simulink model "ideal_forward_converter"  (R2018a)
settings: Solver=FixedStepDiscrete  StartTime=0.0  StopTime=0.01  FixedStep=1e-08  RelTol=1e-3
libraries: powerlib x12, pePowerMeasurement x1
settings Model: Creator=gizemlikaradenizli61  LastModifiedBy=anılcanbudak
settings SolverCC: AlgebraicLoopSolver=LineSearch

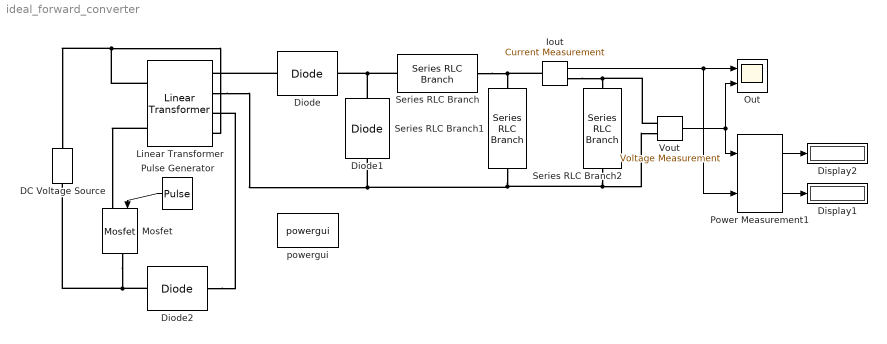
== system ideal_forward_converter ==
  DC Voltage Source : powerlib/Electrical Sources/DC Voltage Source  Amplitude=24  Measurements=None
  Diode : powerlib/Power Electronics/Diode  Ron=0.0001  Lon=0  Vf=0  IC=0  UseSnubber=0  Rs=500  Cs=250e-09  Measurements=off
  Diode1 : powerlib/Power Electronics/Diode  Ron=0.0001  Lon=0  Vf=0  IC=0  UseSnubber=0  Rs=500  Cs=250e-9  Measurements=off
  Diode2 : powerlib/Power Electronics/Diode  Ron=0.001  Lon=0  Vf=0  IC=0  UseSnubber=0  Rs=500  Cs=250e-9  Measurements=off
  Display1 : Display
  Display2 : Display
  Iout : powerlib/Measurements/Current Measurement  PhasorSimulation=off  OutputType=Complex  PSBequivalent=0
  Linear Transformer : powerlib/Elements/Linear Transformer  UNITS=SI  NominalPower=[ 40 30000]  winding1=[32 0.015 0]  winding2=[28.985 0.021 0]  ThreeWindings=on  winding3=[32 0.005 0]  RmLm=[500 0]  Measurements=None  DataType=on
  Mosfet : powerlib/Power Electronics/Mosfet  Ron=0.1  Lon=0  Rd=0.01  Vfd=0  IC=0  Rs=1e05  Cs=inf  Measurements=off
  Out : Scope  NumInputPorts=2
  Power Measurement1 : pePowerMeasurement/Power Measurement  OverrideUsingVariant=Discrete  F=30000  K=[0 1 2 3]  Ts=0.000001
  Pulse Generator : DiscretePulseGenerator  PulseType=Time based  Period=0.000033  PulseWidth=46
  Series RLC Branch : powerlib/Elements/Series RLC Branch  LConnTagsString=__new0  RConnTagsString=__new0  BranchType=L  Resistance=1  Inductance=5e-4  SetiL0=off  InitialCurrent=0  Capacitance=1e-6  Setx0=off  InitialVoltage=0  Measurements=None
  Series RLC Branch1 : powerlib/Elements/Series RLC Branch  LConnTagsString=__new0  RConnTagsString=__new0  BranchType=C  Resistance=1  Inductance=1e-3  SetiL0=off  InitialCurrent=0  Capacitance=10e-6  Setx0=off  InitialVoltage=0  Measurements=None
  Series RLC Branch2 : powerlib/Elements/Series RLC Branch  LConnTagsString=__new0  RConnTagsString=__new0  BranchType=R  Resistance=2.5  Inductance=1e-3  SetiL0=off  InitialCurrent=0  Capacitance=1e-6  Setx0=off  InitialVoltage=0  Measurements=None
  Vout : powerlib/Measurements/Voltage Measurement  PhasorSimulation=off  OutputType=Complex  PSBequivalent=0
  powergui : powerlib/powergui  Priority=1  SimulationMode=Discrete  SampleTime=1e-8  frequency=60  Iterations=50  frequencyindice=0  Pbase=100e6  ErrMax=1e-4  UnitsV=kV  UnitsW=MW  buscounter=0  FunctionMessages=off  echomessages=off  EnableUseOfTLC=off  CurrentSourceSwitches=off  DisableSnubberDevices=off  DisableRonSwitches=off  DisableVfSwitches=off  DisplayEquations=off  SolverType=Tustin/Backward Euler (TBE)  Interpol=off  ExternalGateDelay=off  methode=off  Ts=100  x0status=blocks  SPID=on  SwTol=0  HookPort=off  RestoreLinks=warning  ResistiveCurrentMeasurement=off  Frange=[0:2:500]  Ylog=off  Xlog=on  ShowGrid=off  save=off  variable=ZData  structure=0  ZoomFFT=off  StartTime=0.0  cycles=1  DisplayStyle=1  fundamental=60  FreqAxis=off  MaxFrequency=1000  frequencyindicesteady=1  RmsSteady=1  display=off
  wires:
  Pulse Generator/1 -> Mosfet/1
  Vout/1 -> Out/2, Power Measurement1/1
  Iout/1 -> Out/1, Power Measurement1/2
  Power Measurement1/1 -> Display2/1
  Power Measurement1/2 -> Display1/1
  connections:
  Linear Transformer/LConn2 -- Mosfet/LConn1
  Mosfet/RConn1 -- DC Voltage Source/LConn1 -- Diode2/LConn1
  Series RLC Branch2/RConn1 -- Vout/LConn2 -- Linear Transformer/RConn2 -- Diode1/LConn1 -- Series RLC Branch1/RConn1
  Diode1/RConn1 -- Series RLC Branch/LConn1 -- Diode/RConn1
  Iout/LConn1 -- Series RLC Branch/RConn1 -- Series RLC Branch1/LConn1
  Iout/RConn1 -- Vout/LConn1 -- Series RLC Branch2/LConn1
  Diode/LConn1 -- Linear Transformer/RConn1
  Diode2/RConn1 -- Linear Transformer/RConn3
  Linear Transformer/LConn1 -- DC Voltage Source/RConn1 -- Linear Transformer/RConn4
